simulink library "CTRL_DSI_PedalMap"  (R2023b)
settings: Solver=VariableStepAuto  StartTime=0.0  StopTime=10.0  RelTol=1e-3
settings Model: Creator=blatak  LastModifiedBy=blatak
settings ModelReferenceCC: EnableRefExpFcnMdlSchedulingChecks=on

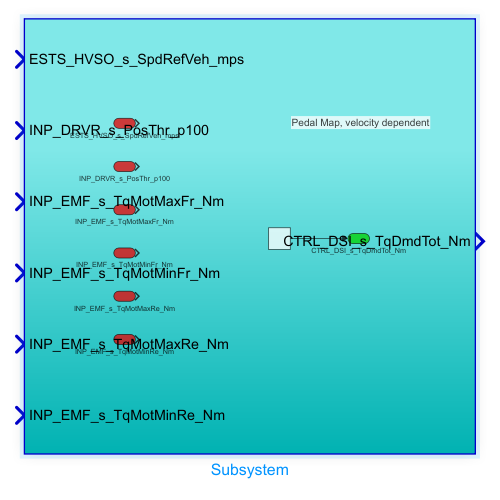
[thumbnail: Simulink's stored preview of the top-level diagram]
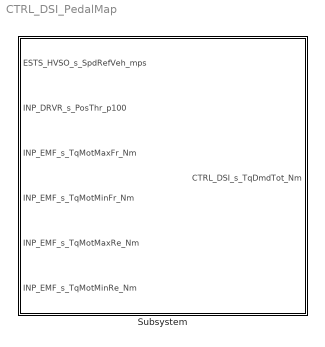
== system CTRL_DSI_PedalMap ==
  Subsystem : Subsystem

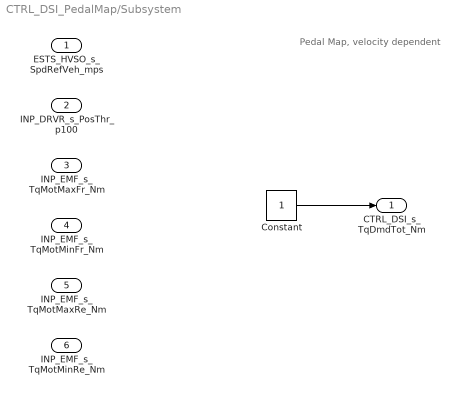
== system CTRL_DSI_PedalMap/Subsystem ==
  note: Pedal Map, velocity dependent
  ESTS_HVSO_s_SpdRefVeh_mps : Inport
  INP_DRVR_s_PosThr_p100 : Inport  Port=2
  INP_EMF_s_TqMotMaxFr_Nm : Inport  Port=3
  INP_EMF_s_TqMotMinFr_Nm : Inport  Port=4
  INP_EMF_s_TqMotMaxRe_Nm : Inport  Port=5
  INP_EMF_s_TqMotMinRe_Nm : Inport  Port=6
  Constant : Constant  OutDataTypeStr=single
  CTRL_DSI_s_TqDmdTot_Nm : Outport
  wires:
  Constant/1 -> CTRL_DSI_s_TqDmdTot_Nm/1
